simulink model "PoLiFirstPrototipe"  (Simulink 7.9)
settings: Solver=ode45  StartTime=0.0  StopTime=10.0  RelTol=1e-3
undefined symbols (not defined in the file or in its folder): sigbuilder_block
settings Model: Creator=lanalfa  LastModifiedBy=lanalfa

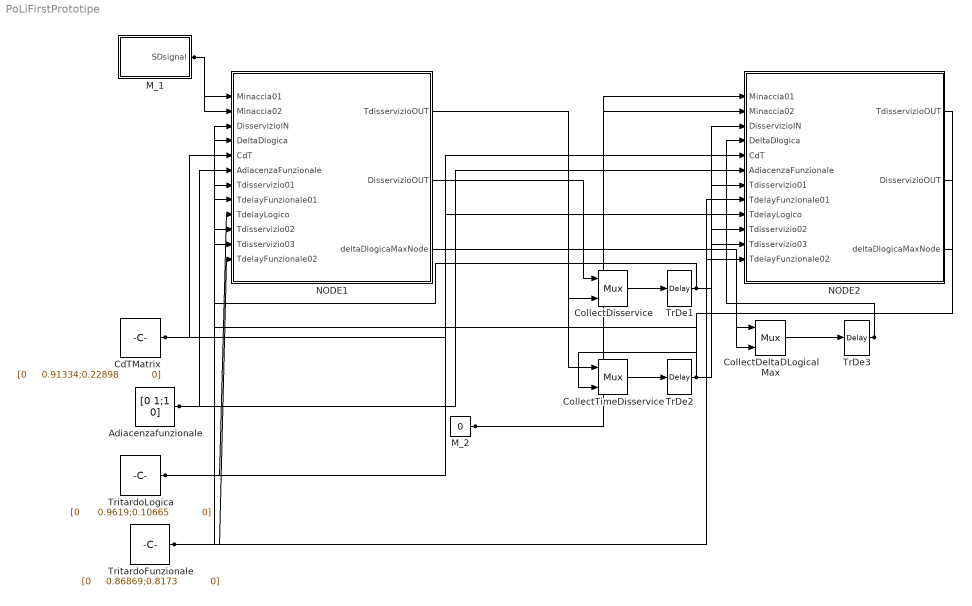
== system PoLiFirstPrototipe ==
  Adiacenzafunzionale : Constant  Value="[0  1;1  0]"
  CdTMatrix : Constant  Value="[0     0.91334;0.22898           0]"
  CollectDeltaDLogicalMax : Mux  Inputs=[-1 -1]
  CollectDisservice : Mux  Inputs=[-1 -1]
  CollectTimeDisservice : Mux  Inputs=[-1 -1]
  M_1 : Subsystem  Tag=STV Subsys  LoadFcn=sigbuilder_block('load');  StartFcn=sigbuilder_block('start');  StopFcn=sigbuilder_block('stop');  ClipboardFcn=sigbuilder_block('clipboard');  mask(Sigbuilder block){}
      mask init:
      | if ~strcmp(get_param(bdroot(gcb),'SimulationStatus'),'stopped'),tuvar = sigbuilder_block('maskInit'); end
      settings: CopyFcn=sigbuilder_block('copy');  DeleteFcn=sigbuilder_block('delete');  ModelCloseFcn=sigbuilder_block('modelClose');  PreSaveFcn=sigbuilder_block('preSave');  NameChangeFcn=sigbuilder_block('namechange');  OpenFcn=sigbuilder_block('open',[50.25 50.25 519.75 399.75 ]);  CloseFcn=sigbuilder_block('close');
      mask Display: plot(0, 0, 100, 100,[2, 2, 32, 32, 2], [68, 8, 8, 68, 68],[32, 2], [38, 38], [32, 19, 2],[53, 60, 44], [32, 17, 17, 2],[16, 16, 31, 31]);txt = getActiveGroup(gcbh);text(2, 100, txt,'verticalAlignment', 'top');
  M_2 : Constant  Value=0
  NODE1 : Subsystem
  NODE2 : Subsystem
  TrDe1 : TransportDelay  DelayTime=0.081472
  TrDe2 : TransportDelay  DelayTime=0.081472
  TrDe3 : TransportDelay  DelayTime=0.081472
  TritardoFunzionale : Constant  Value="[0     0.86869;0.8173           0]"
  TritardoLogica : Constant  Value="[0      0.9619;0.10665           0]"
  wires:
  M_1/1(SDsignal) -> NODE1/1(Minaccia01), NODE1/2(Minaccia02)
  M_2/1 -> NODE2/1(Minaccia01), NODE2/2(Minaccia02)
  CollectDisservice/1 -> TrDe1/1
  CollectTimeDisservice/1 -> TrDe2/1
  CollectDeltaDLogicalMax/1 -> TrDe3/1
  CdTMatrix/1 -> NODE1/5(CdT), NODE2/5(CdT)
  Adiacenzafunzionale/1 -> NODE1/6(AdiacenzaFunzionale), NODE2/6(AdiacenzaFunzionale)
  TritardoLogica/1 -> NODE1/9(TdelayLogico), NODE2/9(TdelayLogico)
  TritardoFunzionale/1 -> NODE1/8(TdelayFunzionale01), NODE1/12(TdelayFunzionale02), NODE2/8(TdelayFunzionale01), NODE2/12(TdelayFunzionale02)
  TrDe1/1 -> NODE1/3(DisservizioIN), NODE2/3(DisservizioIN)
  TrDe2/1 -> NODE1/7(Tdisservizio01), NODE1/10(Tdisservizio02), NODE1/11(Tdisservizio03), NODE2/7(Tdisservizio01), NODE2/10(Tdisservizio02), NODE2/11(Tdisservizio03)
  TrDe3/1 -> NODE1/4(DeltaDlogica), NODE2/4(DeltaDlogica)
  NODE1/1(TdisservizioOUT) -> CollectTimeDisservice/1
  NODE1/2(DisservizioOUT) -> CollectDisservice/1
  NODE1/3(deltaDlogicaMaxNode) -> CollectDeltaDLogicalMax/1
  NODE2/1(TdisservizioOUT) -> CollectTimeDisservice/2
  NODE2/2(DisservizioOUT) -> CollectDisservice/2
  NODE2/3(deltaDlogicaMaxNode) -> CollectDeltaDLogicalMax/2

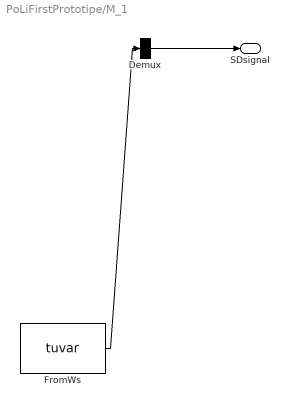
== system PoLiFirstPrototipe/M_1 ==
  Demux : Demux  Tag=STV Demux  Outputs=1
  FromWs : FromWorkspace  Tag=STV FromWs  VariableName=tuvar  SampleTime=0  SigBuilderData=DataTag0  VnvData=DataTag1
      SigBuilderData=|
      | dataSet.timeRange = [0 24]
      | dataSet.name = 'Group 1'
      | sbobj.Name = 'Signal Builder'
      | sbobj.Groups.Name = 'Group 1'
      | sbobj.Groups.Signals.Name = 'SDsignal'
      | sbobj.Groups.Signals.XData = [0 1 1 4 4 8 8 10 10 24]
      | sbobj.Groups.Signals.YData = [0 0 1 1 0 0 0.5 0.5 0 0]
      | sbobj.Groups.TimeRange = [0 24]
  SDsignal : Outport  Tag=STV Outport
  wires:
  FromWs/1 -> Demux/1
  Demux/1 -> SDsignal/1

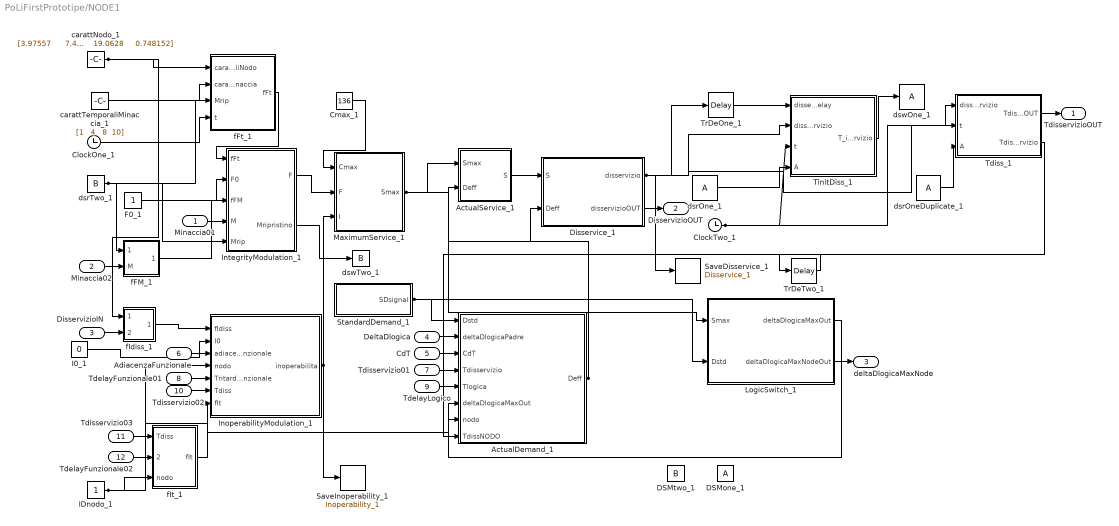
== system PoLiFirstPrototipe/NODE1 ==
  Minaccia01 : Inport
  Minaccia02 : Inport  Port=2
  DisservizioIN : Inport  Port=3
  DeltaDlogica : Inport  Port=4
  CdT : Inport  Port=5
  AdiacenzaFunzionale : Inport  Port=6
  Tdisservizio01 : Inport  Port=7
  TdelayFunzionale01 : Inport  Port=8
  TdelayLogico : Inport  Port=9
  Tdisservizio02 : Inport  Port=10
  Tdisservizio03 : Inport  Port=11
  TdelayFunzionale02 : Inport  Port=12
  ActualDemand_1 : MATLAB Function  TreatAsAtomicUnit=on
  ActualService_1 : MATLAB Function  TreatAsAtomicUnit=on
  ClockOne_1 : Clock
  ClockTwo_1 : Clock
  Cmax_1 : Constant  Value=136
  DSMone_1 : DataStoreMemory
  DSMtwo_1 : DataStoreMemory  DataStoreName=B
  Disservice_1 : MATLAB Function  TreatAsAtomicUnit=on
  F0_1 : Constant
  I0_1 : Constant  Value=0
  IDnodo_1 : Constant
  InoperabilityModulation_1 : MATLAB Function  TreatAsAtomicUnit=on
  IntegrityModulation_1 : MATLAB Function  TreatAsAtomicUnit=on
  LogicSwitch_1 : MATLAB Function  TreatAsAtomicUnit=on
  MaximumService_1 : MATLAB Function  TreatAsAtomicUnit=on
  SaveDisservice_1 : ToWorkspace  VariableName=Disservice_1  SampleTime=-1
  SaveInoperability_1 : ToWorkspace  VariableName=Inoperability_1  SampleTime=-1
  StandardDemand_1 : Subsystem  Tag=STV Subsys  LoadFcn=sigbuilder_block('load');  StartFcn=sigbuilder_block('start');  StopFcn=sigbuilder_block('stop');  ClipboardFcn=sigbuilder_block('clipboard');  mask(Sigbuilder block){}
      mask init:
      | if ~strcmp(get_param(bdroot(gcb),'SimulationStatus'),'stopped'),tuvar = sigbuilder_block('maskInit'); end
      settings: CopyFcn=sigbuilder_block('copy');  DeleteFcn=sigbuilder_block('delete');  ModelCloseFcn=sigbuilder_block('modelClose');  PreSaveFcn=sigbuilder_block('preSave');  NameChangeFcn=sigbuilder_block('namechange');  OpenFcn=sigbuilder_block('open',[50.25 50.25 519.75 399.75 ]);  CloseFcn=sigbuilder_block('close');
      mask Display: plot(0, 0, 100, 100,[2, 2, 32, 32, 2], [68, 8, 8, 68, 68],[32, 2], [38, 38], [32, 19, 2],[53, 60, 44], [32, 17, 17, 2],[16, 16, 31, 31]);txt = getActiveGroup(gcbh);text(2, 100, txt,'verticalAlignment', 'top');
  Tdiss_1 : MATLAB Function  TreatAsAtomicUnit=on
  TinitDiss_1 : MATLAB Function  TreatAsAtomicUnit=on
  TrDeOne_1 : TransportDelay  DelayTime=0.081472
  TrDeTwo_1 : TransportDelay  DelayTime=0.081472
  carattNodo_1 : Constant  Value="[3.97557      7.46916      12.6848      19.0628     0.748152]"
  carattTemporaliMinaccia_1 : Constant  Value="[1   4   8  10]"
  dsrOneDuplicate_1 : DataStoreRead
  dsrOne_1 : DataStoreRead
  dsrTwo_1 : DataStoreRead  DataStoreName=B
  dswOne_1 : DataStoreWrite
  dswTwo_1 : DataStoreWrite  DataStoreName=B
  fFM_1 : MATLAB Function  TreatAsAtomicUnit=on
  fFt_1 : MATLAB Function  TreatAsAtomicUnit=on
  fIdiss_1 : MATLAB Function  TreatAsAtomicUnit=on
  fIt_1 : MATLAB Function  TreatAsAtomicUnit=on
  TdisservizioOUT : Outport
  DisservizioOUT : Outport  Port=2
  deltaDlogicaMaxNode : Outport  Port=3
  wires:
  carattNodo_1/1 -> fFt_1/1(carattTemporaliNodo), fIdiss_1/1(parameters)
  carattTemporaliMinaccia_1/1 -> fFt_1/2(carattTemporaliMinaccia)
  ClockOne_1/1 -> fFt_1/4(t)
  fFt_1/1(fFt) -> IntegrityModulation_1/1(fFt)
  dsrTwo_1/1 -> fFt_1/3(Mrip), IntegrityModulation_1/5(Mrip), fFM_1/1(Mrip)
  F0_1/1 -> IntegrityModulation_1/2(F0)
  fFM_1/1(fFM) -> IntegrityModulation_1/3(fFM)
  IntegrityModulation_1/1(F) -> MaximumService_1/2(F)
  IntegrityModulation_1/2(Mripristino) -> dswTwo_1/1
  MaximumService_1/1(Smax) -> ActualService_1/1(Smax), LogicSwitch_1/1(Smax)
  Cmax_1/1 -> MaximumService_1/1(Cmax)
  ActualService_1/1(S) -> Disservice_1/1(S)
  Disservice_1/1(disservizio) -> TinitDiss_1/2(disservizio), Tdiss_1/1(disservizio), TrDeOne_1/1, SaveDisservice_1/1
  TinitDiss_1/1(T_inizio_disservizio) -> dswOne_1/1
  Tdiss_1/2(Tdisservizio) -> TrDeTwo_1/1
  TrDeOne_1/1 -> TinitDiss_1/1(disservizioDelay)
  ClockTwo_1/1 -> TinitDiss_1/3(t), Tdiss_1/2(t)
  dsrOne_1/1 -> TinitDiss_1/4(A)
  dsrOneDuplicate_1/1 -> Tdiss_1/3(A)
  InoperabilityModulation_1/1(inoperabilita) -> MaximumService_1/3(I), SaveInoperability_1/1
  ActualDemand_1/1(Deff) -> ActualService_1/2(Deff), Disservice_1/2(Deff)
  LogicSwitch_1/1(deltaDlogicaMaxOut) -> ActualDemand_1/6(deltaDlogicaMaxOut)
  fIdiss_1/1(fIdiss) -> InoperabilityModulation_1/1(fIdiss)
  I0_1/1 -> InoperabilityModulation_1/2(I0)
  fIt_1/1(fIt) -> InoperabilityModulation_1/7(fIt)
  IDnodo_1/1 -> InoperabilityModulation_1/4(nodo), ActualDemand_1/7(nodo), fIt_1/3(nodo)
  StandardDemand_1/1(SDsignal) -> ActualDemand_1/1(Dstd), LogicSwitch_1/2(Dstd)
  TrDeTwo_1/1 -> ActualDemand_1/8(TdissNODO)
  Tdiss_1/1(TdisservizioOUT) -> TdisservizioOUT/1
  Disservice_1/2(disservizioOUT) -> DisservizioOUT/1
  Minaccia01/1 -> IntegrityModulation_1/4(M)
  Minaccia02/1 -> fFM_1/2(M)
  DisservizioIN/1 -> fIdiss_1/2(DisservizioIN)
  DeltaDlogica/1 -> ActualDemand_1/2(deltaDlogicaPadre)
  CdT/1 -> ActualDemand_1/3(CdT)
  AdiacenzaFunzionale/1 -> InoperabilityModulation_1/3(adiacenzaFunzionale)
  LogicSwitch_1/2(deltaDlogicaMaxNodeOut) -> deltaDlogicaMaxNode/1
  Tdisservizio01/1 -> ActualDemand_1/4(Tdisservizio)
  TdelayFunzionale01/1 -> InoperabilityModulation_1/5(TritardoFunzionale)
  TdelayLogico/1 -> ActualDemand_1/5(Tlogica)
  Tdisservizio02/1 -> InoperabilityModulation_1/6(Tdiss)
  Tdisservizio03/1 -> fIt_1/1(Tdiss)
  TdelayFunzionale02/1 -> fIt_1/2(TritardoFunzionale)

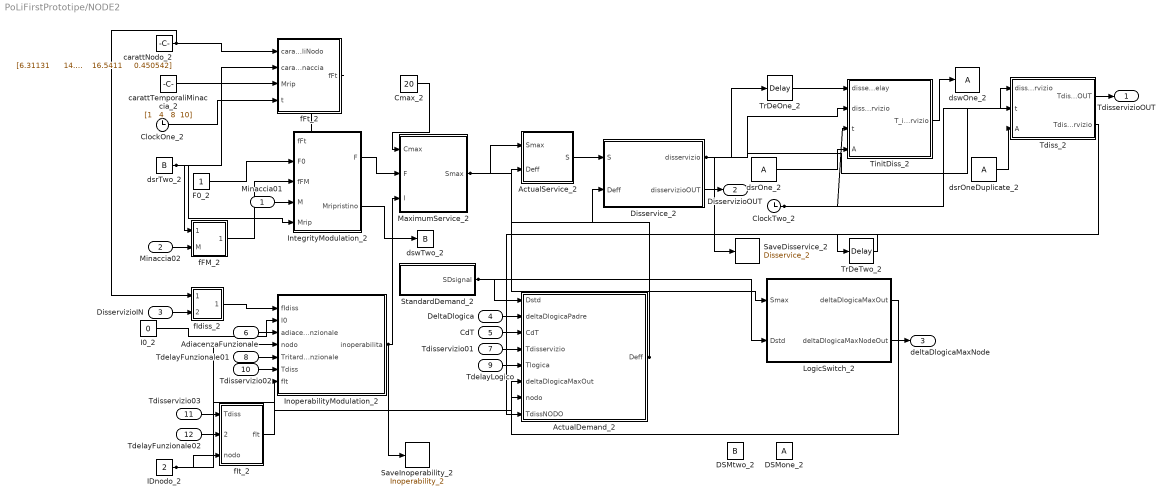
== system PoLiFirstPrototipe/NODE2 ==
  Minaccia01 : Inport
  Minaccia02 : Inport  Port=2
  DisservizioIN : Inport  Port=3
  DeltaDlogica : Inport  Port=4
  CdT : Inport  Port=5
  AdiacenzaFunzionale : Inport  Port=6
  Tdisservizio01 : Inport  Port=7
  TdelayFunzionale01 : Inport  Port=8
  TdelayLogico : Inport  Port=9
  Tdisservizio02 : Inport  Port=10
  Tdisservizio03 : Inport  Port=11
  TdelayFunzionale02 : Inport  Port=12
  ActualDemand_2 : MATLAB Function  TreatAsAtomicUnit=on
  ActualService_2 : MATLAB Function  TreatAsAtomicUnit=on
  ClockOne_2 : Clock
  ClockTwo_2 : Clock
  Cmax_2 : Constant  Value=20
  DSMone_2 : DataStoreMemory
  DSMtwo_2 : DataStoreMemory  DataStoreName=B
  Disservice_2 : MATLAB Function  TreatAsAtomicUnit=on
  F0_2 : Constant
  I0_2 : Constant  Value=0
  IDnodo_2 : Constant  Value=2
  InoperabilityModulation_2 : MATLAB Function  TreatAsAtomicUnit=on
  IntegrityModulation_2 : MATLAB Function  TreatAsAtomicUnit=on
  LogicSwitch_2 : MATLAB Function  TreatAsAtomicUnit=on
  MaximumService_2 : MATLAB Function  TreatAsAtomicUnit=on
  SaveDisservice_2 : ToWorkspace  VariableName=Disservice_2  SampleTime=-1
  SaveInoperability_2 : ToWorkspace  VariableName=Inoperability_2  SampleTime=-1
  StandardDemand_2 : Subsystem  Tag=STV Subsys  LoadFcn=sigbuilder_block('load');  StartFcn=sigbuilder_block('start');  StopFcn=sigbuilder_block('stop');  ClipboardFcn=sigbuilder_block('clipboard');  mask(Sigbuilder block){}
      mask init:
      | if ~strcmp(get_param(bdroot(gcb),'SimulationStatus'),'stopped'),tuvar = sigbuilder_block('maskInit'); end
      settings: CopyFcn=sigbuilder_block('copy');  DeleteFcn=sigbuilder_block('delete');  ModelCloseFcn=sigbuilder_block('modelClose');  PreSaveFcn=sigbuilder_block('preSave');  NameChangeFcn=sigbuilder_block('namechange');  OpenFcn=sigbuilder_block('open',[50.25 50.25 519.75 399.75 ]);  CloseFcn=sigbuilder_block('close');
      mask Display: plot(0, 0, 100, 100,[2, 2, 32, 32, 2], [68, 8, 8, 68, 68],[32, 2], [38, 38], [32, 19, 2],[53, 60, 44], [32, 17, 17, 2],[16, 16, 31, 31]);txt = getActiveGroup(gcbh);text(2, 100, txt,'verticalAlignment', 'top');
  Tdiss_2 : MATLAB Function  TreatAsAtomicUnit=on
  TinitDiss_2 : MATLAB Function  TreatAsAtomicUnit=on
  TrDeOne_2 : TransportDelay  DelayTime=0.081472
  TrDeTwo_2 : TransportDelay  DelayTime=0.081472
  carattNodo_2 : Constant  Value="[6.31131      14.4476      15.6979      16.5411     0.450542]"
  carattTemporaliMinaccia_2 : Constant  Value="[1   4   8  10]"
  dsrOneDuplicate_2 : DataStoreRead
  dsrOne_2 : DataStoreRead
  dsrTwo_2 : DataStoreRead  DataStoreName=B
  dswOne_2 : DataStoreWrite
  dswTwo_2 : DataStoreWrite  DataStoreName=B
  fFM_2 : MATLAB Function  TreatAsAtomicUnit=on
  fFt_2 : MATLAB Function  TreatAsAtomicUnit=on
  fIdiss_2 : MATLAB Function  TreatAsAtomicUnit=on
  fIt_2 : MATLAB Function  TreatAsAtomicUnit=on
  TdisservizioOUT : Outport
  DisservizioOUT : Outport  Port=2
  deltaDlogicaMaxNode : Outport  Port=3
  wires:
  carattNodo_2/1 -> fFt_2/1(carattTemporaliNodo), fIdiss_2/1(parameters)
  carattTemporaliMinaccia_2/1 -> fFt_2/2(carattTemporaliMinaccia)
  ClockOne_2/1 -> fFt_2/4(t)
  fFt_2/1(fFt) -> IntegrityModulation_2/1(fFt)
  dsrTwo_2/1 -> fFt_2/3(Mrip), IntegrityModulation_2/5(Mrip), fFM_2/1(Mrip)
  F0_2/1 -> IntegrityModulation_2/2(F0)
  fFM_2/1(fFM) -> IntegrityModulation_2/3(fFM)
  IntegrityModulation_2/1(F) -> MaximumService_2/2(F)
  IntegrityModulation_2/2(Mripristino) -> dswTwo_2/1
  MaximumService_2/1(Smax) -> ActualService_2/1(Smax), LogicSwitch_2/1(Smax)
  Cmax_2/1 -> MaximumService_2/1(Cmax)
  ActualService_2/1(S) -> Disservice_2/1(S)
  Disservice_2/1(disservizio) -> TinitDiss_2/2(disservizio), Tdiss_2/1(disservizio), TrDeOne_2/1, SaveDisservice_2/1
  TinitDiss_2/1(T_inizio_disservizio) -> dswOne_2/1
  Tdiss_2/2(Tdisservizio) -> TrDeTwo_2/1
  TrDeOne_2/1 -> TinitDiss_2/1(disservizioDelay)
  ClockTwo_2/1 -> TinitDiss_2/3(t), Tdiss_2/2(t)
  dsrOne_2/1 -> TinitDiss_2/4(A)
  dsrOneDuplicate_2/1 -> Tdiss_2/3(A)
  InoperabilityModulation_2/1(inoperabilita) -> MaximumService_2/3(I), SaveInoperability_2/1
  ActualDemand_2/1(Deff) -> ActualService_2/2(Deff), Disservice_2/2(Deff)
  LogicSwitch_2/1(deltaDlogicaMaxOut) -> ActualDemand_2/6(deltaDlogicaMaxOut)
  fIdiss_2/1(fIdiss) -> InoperabilityModulation_2/1(fIdiss)
  I0_2/1 -> InoperabilityModulation_2/2(I0)
  fIt_2/1(fIt) -> InoperabilityModulation_2/7(fIt)
  IDnodo_2/1 -> InoperabilityModulation_2/4(nodo), ActualDemand_2/7(nodo), fIt_2/3(nodo)
  StandardDemand_2/1(SDsignal) -> ActualDemand_2/1(Dstd), LogicSwitch_2/2(Dstd)
  TrDeTwo_2/1 -> ActualDemand_2/8(TdissNODO)
  Tdiss_2/1(TdisservizioOUT) -> TdisservizioOUT/1
  Disservice_2/2(disservizioOUT) -> DisservizioOUT/1
  Minaccia01/1 -> IntegrityModulation_2/4(M)
  Minaccia02/1 -> fFM_2/2(M)
  DisservizioIN/1 -> fIdiss_2/2(DisservizioIN)
  DeltaDlogica/1 -> ActualDemand_2/2(deltaDlogicaPadre)
  CdT/1 -> ActualDemand_2/3(CdT)
  AdiacenzaFunzionale/1 -> InoperabilityModulation_2/3(adiacenzaFunzionale)
  LogicSwitch_2/2(deltaDlogicaMaxNodeOut) -> deltaDlogicaMaxNode/1
  Tdisservizio01/1 -> ActualDemand_2/4(Tdisservizio)
  TdelayFunzionale01/1 -> InoperabilityModulation_2/5(TritardoFunzionale)
  TdelayLogico/1 -> ActualDemand_2/5(Tlogica)
  Tdisservizio02/1 -> InoperabilityModulation_2/6(Tdiss)
  Tdisservizio03/1 -> fIt_2/1(Tdiss)
  TdelayFunzionale02/1 -> fIt_2/2(TritardoFunzionale)

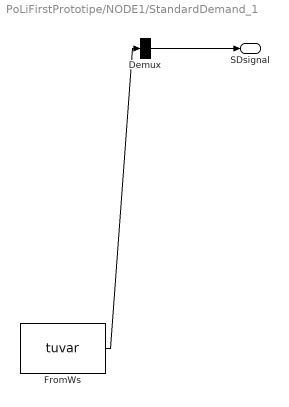
== system PoLiFirstPrototipe/NODE1/StandardDemand_1 ==
  Demux : Demux  Tag=STV Demux  Outputs=1
  FromWs : FromWorkspace  Tag=STV FromWs  VariableName=tuvar  SampleTime=0  SigBuilderData=DataTag2  VnvData=DataTag3
      SigBuilderData=|
      | dataSet.timeRange = [0 24]
      | dataSet.name = 'Group 1'
      | sbobj.Name = 'Signal Builder'
      | sbobj.Groups.Name = 'Group 1'
      | sbobj.Groups.Signals.Name = 'SDsignal'
      | sbobj.Groups.Signals.XData = [0 0.5 1 1.5 2 2.5 3 3.5 4 4.5 5 5.5 6 6.5 7 7.5 8 8.5 9 9.5 10 10.5 11 11.5 12 12.5 13 13.5 14 14.5 15 15.5 16 16.5 17 17.5 18 18.5 19 19.5 20 20.5 21 21.5 22 22.5 23 23.5 24]
      | sbobj.Groups.Signals.YData = [11.7808835651 122.73450492 61.6241133881 4.7751592129 3.99938168056 69.9889117737 116.703457947 11.4599685743 5.50903001057 131.143211714 8.97691830497 32.9473422413 82.6571253434 112.718610458 131.670732893 129.720690874 24.0097353475 92.8744707117 131.315333052 84.1080498354 27.8528134454 69.3920421728 48.1014306249 33.3626112504 43.5604359479 113.884804014 68.2224889304 89.7075411734 105.561576229 101.307064298 40.9255657187 5.53636617206 117.147075775 100.978877439 101.41762366 102.880604253 88.4022078261 101.852595315 71.6327165492 23.0073066061 61.2375892724 97.1258934404 33.4928431781 58.7762568614 128.662783861 30.0332567061 118.332755648 72.1628728161 90.1513203618]
      | sbobj.Groups.TimeRange = [0 24]
  SDsignal : Outport  Tag=STV Outport
  wires:
  FromWs/1 -> Demux/1
  Demux/1 -> SDsignal/1

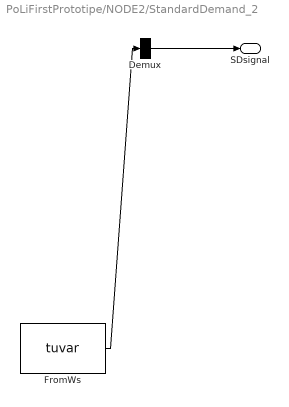
== system PoLiFirstPrototipe/NODE2/StandardDemand_2 ==
  Demux : Demux  Tag=STV Demux  Outputs=1
  FromWs : FromWorkspace  Tag=STV FromWs  VariableName=tuvar  SampleTime=0  SigBuilderData=DataTag4  VnvData=DataTag5
      SigBuilderData=|
      | dataSet.timeRange = [0 24]
      | dataSet.name = 'Group 1'
      | sbobj.Name = 'Signal Builder'
      | sbobj.Groups.Name = 'Group 1'
      | sbobj.Groups.Signals.Name = 'SDsignal'
      | sbobj.Groups.Signals.XData = [0 0.5 1 1.5 2 2.5 3 3.5 4 4.5 5 5.5 6 6.5 7 7.5 8 8.5 9 9.5 10 10.5 11 11.5 12 12.5 13 13.5 14 14.5 15 15.5 16 16.5 17 17.5 18 18.5 19 19.5 20 20.5 21 21.5 22 22.5 23 23.5 24]
      | sbobj.Groups.Signals.YData = [7.35281507549 14.4300356227 0.849863291314 16.8477383664 0.856661035141 3.99439062222 11.5647743475 4.15585340881 6.88518601687 3.01741388262 6.42529690284 5.1373506375 6.89044219645 5.87907823961 14.4615403008 18.0573643753 6.10342754048 0.995559023233 11.2251128069 4.68966423702 16.2625479089 11.0882759858 5.81270338284 14.47949846 6.89803992052 17.6200463688 0.805120829678 8.2946449804 4.97465881389 9.8808589667 2.18193494928 9.05568940072 17.0141198888 3.18565488033 3.71430347862 1.41472753626 16.0680949914 7.67910647707 12.9668098587 8.29471817695 1.6561267234 4.85599541779 12.3910830605 18.4829142087 9.38404893982 1.31978631542 8.62352678256 19.76195861 16.7563538361]
      | sbobj.Groups.TimeRange = [0 24]
  SDsignal : Outport  Tag=STV Outport
  wires:
  FromWs/1 -> Demux/1
  Demux/1 -> SDsignal/1

== matlab function NODE1/fFM_1 ==
  data: Mrip input double; fFM output double; M input double
function fFM = f(Mrip,M)

% Function description:

% This function ....

% INPUT
% ...

% OUTPUT
% ...



%Funzione di modulazione dell'integrità funzionale in intensità retta con coefficiente=1
fFM=[0,0];
fFM(1)=M*1; %modulazione in intensità, %modulazione in intesità della minaccia FM=[0 a 1]
fFM(2)=Mrip*1; %modulazione in intensità, da usare solo per il recupero di integrità,cioè quando M=0;

== matlab function NODE1/fFt_1 ==
  data: carattTemporaliNodo input double; fFt output double; carattTemporaliMinaccia input double; Mrip input double; t input double
function fFt = f(carattTemporaliNodo,carattTemporaliMinaccia,Mrip,t)

% Function description:

% This function ....

% INPUT
% ...

% OUTPUT
% ...

%Funzione di modulazione dell'integrità funzionale nel tempo, nel caso di
%due minaccie differenti per inizio attacco nel tempo.

Tbuffer=carattTemporaliNodo(1);
Tpropagazione=carattTemporaliNodo(2);
TorganizzazioneMax=carattTemporaliNodo(3);
TripristinoMax=carattTemporaliNodo(4);
TinizioM1=carattTemporaliMinaccia(1);  %da impostare manualmente nelle descrizione minaccia
TfineM1=carattTemporaliMinaccia(2); %da impostare manualmente nelle descrizione minaccia
TinizioM2=carattTemporaliMinaccia(3); %da impostare manualmente nelle descrizione minaccia
TfineM2=carattTemporaliMinaccia(4); %da impostare manualmente nelle descrizione minaccia
Torganizzazione=Mrip*TorganizzazioneMax;
Tripristino=TripristinoMax*Mrip; %in realtà sarebbe Tripristino=TripristinoMax*M; ma così M mi annulla il ripristino a fine minaccia, uso minaccia salvata  
tauRipristino=Tripristino/5; %controllare se vale anche per nodo non trasporto
tauPropagazione=Tpropagazione/5; %controllare se vale anche per nodo non trasporto
t0=TinizioM1+Tbuffer;
t1=t0+Tpropagazione;
t2o=t1+Torganizzazione;
t2m=TfineM1;
if t2m>=t2o %chiarire cosa succede se M=0 ma non ancora organizzato (t2o>t2m) e quindi cosa fa integrità funzionale
    t2=t2m;
else t2=t2o;
end
t3=t2+Tripristino;
t4=TinizioM2+Tbuffer;
t5=t4+Tpropagazione;
t6m=TfineM2;
t6o=t5+Torganizzazione; 
if t6m>=t6o
    t6=t6m;
else t6=t6o;
end
t7=t6+Tripristino;

if t<t0
    fFt=0;
elseif t>=t0 && t<t1 
        fFt=1-exp(-(t-t0)/tauPropagazione);
elseif t>=t1 && t<t2
        fFt=1;
elseif t>=t2 && t<t3 
        fFt=exp(-(t-t2)/tauRipristino);  
elseif t>=t4 && t<t5
        fFt=1-exp(-(t-t4)/tauPropagazione);
elseif t>=t5 && t<t6
        fFt=1;
elseif t>=t6 && t<t7
        fFt=exp(-(t-t6)/tauRipristino);  
else fFt=0;
end

== matlab function NODE1/IntegrityModulation_1 ==
  data: fFt input double; F output double; F0 input double; fFM input double; M input double; Mrip input double; Mripristino output double
function [F,Mripristino] = f(fFt,F0,fFM,M,Mrip)

% Function description:

% This function ....

% INPUT
% ...

% OUTPUT
% ...


% Codice con valutazione solo in intesità, non nel tempo.
% fFM=M*FM; %modulazione in intensità
% fFt=1;
% i=F0-fFM*fFt;
%
% if i<0
%     F=0;
% else
%     F=i;
% end

% Codice con valutazione in intensità e tempo con doppia attacco da parte della minaccia

% Modifica per avere ripristino a fine minaccia, in realtà sarebbe sempre i=F0-fFM*fFt

if M>0
    i=F0-fFM(1)*fFt;
    Mripristino=M;
else i=F0-fFM(2)*fFt; %fFM(2) è quella usata solo per il ripristino di integrità perchè M=0;
    Mripristino=Mrip;
end

if i<0
    F=0;
else
    F=i;
end

== matlab function NODE1/MaximumService_1 ==
  data: Cmax input double; Smax output double; F input double; I input double
function Smax = f(Cmax,F,I)

% Function description:

% This function ....

% INPUT
% ...

% OUTPUT
% ...


Smax=F*(1-I)*Cmax;

end

== matlab function NODE1/ActualService_1 ==
  data: Smax input double; S output double; Deff input double
function S = f(Smax,Deff)

% Function description:

% This function ....

% INPUT
% ...

% OUTPUT
% ...

if Deff>Smax
    S=Smax;
else
    S=Deff;
end

== matlab function NODE1/Disservice_1 ==
  data: S input double; disservizio output double; Deff input double; disservizioOUT output double
function [disservizio,disservizioOUT ] = f(S,Deff)

% Function description:

% This function ....

% INPUT
% ...

% OUTPUT
% ...

if Deff==0
    disservizio=0;
else
disservizio=(Deff-S)/Deff;

end

disservizioOUT=disservizio;

== matlab function NODE1/TinitDiss_1 ==
  data: disservizioDelay input double; T_inizio_disservizio output double; disservizio input double; t input double; A input double
function T_inizio_disservizio  = f(disservizioDelay,disservizio,t,A)

% Function description:

% This function ....

% INPUT
% ...

% OUTPUT
% ...

if disservizioDelay==0 && disservizio>0
    T_inizio_disservizio=t;
else T_inizio_disservizio=A;

end

% if disservizioDelay~=disservizio && disservizio>0
%     T_inizio_variazioneDiss=t;
% else T_inizio_variazioneDiss=B;
% end
%

== matlab function NODE1/Tdiss_1 ==
  data: disservizio input double; TdisservizioOUT output double; t input double; A input double; Tdisservizio output double
function [TdisservizioOUT,Tdisservizio]  = f(disservizio,t,A)

% Function description:

% This function ....

% INPUT
% ...

% OUTPUT
% ...


if disservizio==0
    Tdisservizio=0;
else
    Tdisservizio=t-A;
end
% if disservizio==0
%     TvariazioneDiss=0;
% else
%     TvariazioneDiss=t-B;
% end

TdisservizioOUT=Tdisservizio;

== matlab function NODE1/InoperabilityModulation_1 ==
  data: fIdiss input double; inoperabilita output double; I0 input double; adiacenzaFunzionale input double; nodo input double; TritardoFunzionale input double; Tdiss input double; fIt input double
function inoperabilita = f(fIdiss,I0,adiacenzaFunzionale,nodo,TritardoFunzionale,Tdiss,fIt)

% Function description:

% This function ....

% INPUT
% ...

% OUTPUT
% ...


j=1;
disservizioTot=zeros(length(adiacenzaFunzionale),1);
for j=1:length(adiacenzaFunzionale)
    if adiacenzaFunzionale(j,nodo)==1 && Tdiss(j)>=TritardoFunzionale(j,nodo)
        disservizioTot(j,1)=fIdiss(1,j)*fIt(1,j);
        %disservizioTot(j,1)=fIdiss; se non voglio avere
        %modulazione nel tempo del trasferimento di disservizio in
        %inoperabilità
    else disservizioTot(j,1)=0;
    end
end

disservizioTotIN=sum(disservizioTot); % ho fatto somma, altro approccio prendere il max
i=I0+disservizioTotIN;

if i>1
    inoperabilita=1;
elseif i<=0
    inoperabilita=0;
else inoperabilita=i;
end

== matlab function NODE1/ActualDemand_1 ==
  data: Dstd input double; Deff output double; deltaDlogicaPadre input double; CdT input double; Tdisservizio input double; Tlogica input double; deltaDlogicaMaxOut input double; nodo input double; TdissNODO input double
function Deff= f(Dstd,deltaDlogicaPadre,CdT,Tdisservizio,Tlogica,deltaDlogicaMaxOut,nodo,TdissNODO)
 
% Function description:
 
% This function ....
 
% INPUT
% ...
 
% OUTPUT
% ...
 
 
j=1;
deltaDlogicaOUT=zeros(length(CdT),1);
deltaDlogicaIN=zeros(length(CdT),1);
 
 
for j=1:(length(CdT))
    if Tdisservizio(j)>=Tlogica(j,nodo) && CdT(j,nodo)>0
        deltaDlogicaIN(j,1)=CdT(j,nodo)*deltaDlogicaPadre(j);
    else
        deltaDlogicaIN(j,1)=0;
    end
    if TdissNODO>=Tlogica(nodo,j) && CdT(nodo,j)>0
          deltaDlogicaOUT(j,1)=CdT(nodo,j)*deltaDlogicaMaxOut;
    else
        deltaDlogicaOUT(j,1)=0;
    end
end
deltaDlogicaTotIN=sum(deltaDlogicaIN);
deltaDlogicaTotOut=sum(deltaDlogicaOUT);
 
 
Deff=Dstd+deltaDlogicaTotIN-deltaDlogicaTotOut;

== matlab function NODE1/LogicSwitch_1 ==
  data: Smax input double; deltaDlogicaMaxOut output double; Dstd input double; deltaDlogicaMaxNodeOut output double
function [deltaDlogicaMaxOut,deltaDlogicaMaxNodeOut] = f(Smax,Dstd)

% Function description:

% This function ....

% INPUT
% ...

% OUTPUT
% ...

deltaDlogicaMaxOut=Dstd-Smax;
if deltaDlogicaMaxOut<0
    deltaDlogicaMaxOut=0;
end

deltaDlogicaMaxNodeOut=deltaDlogicaMaxOut;

== matlab function NODE1/fIdiss_1 ==
  data: parameters input double; fIdiss output double; DisservizioIN input double
function fIdiss = f(parameters,DisservizioIN)

% Function description:

% This function ....

% INPUT
% ...

% OUTPUT
% ...


%Funzione di modulazion lineare con coefficiente angolare variabile,
fIdiss=zeros(1,length(DisservizioIN));
j=1;
for j=1:length(DisservizioIN)
    fIdiss(1,j)=DisservizioIN(j)*parameters(5);% modulazione in intensità
end

== matlab function NODE1/fIt_1 ==
  data: Tdiss input double; fIt output double; TritardoFunzionale input double; nodo input double
function fIt = f(Tdiss,TritardoFunzionale,nodo)

% Function description:

% This function ....

% INPUT
% ...

% OUTPUT
% ...

%funzione di modulazione dell'inoperabilità nel tempo
fIt=zeros(1,length(Tdiss));
j=1;
for j=1:length(Tdiss)
    tau=TritardoFunzionale(j,nodo)/5; %vedere se anche per i nodi non di trasporto vale questa tau!!!
    fIt(1,j)=1-exp(-(Tdiss(j)-TritardoFunzionale(j,nodo))/tau);%modulazione nel tempo
end

== matlab function NODE2/fFt_2 ==
  data: carattTemporaliNodo input double; fFt output double; carattTemporaliMinaccia input double; Mrip input double; t input double
function fFt = f(carattTemporaliNodo,carattTemporaliMinaccia,Mrip,t)

% Function description:

% This function ....

% INPUT
% ...

% OUTPUT
% ...

%Funzione di modulazione dell'integrità funzionale nel tempo, nel caso di
%due minaccie differenti per inizio attacco nel tempo.

Tbuffer=carattTemporaliNodo(1);
Tpropagazione=carattTemporaliNodo(2);
TorganizzazioneMax=carattTemporaliNodo(3);
TripristinoMax=carattTemporaliNodo(4);
TinizioM1=carattTemporaliMinaccia(1);  %da impostare manualmente nelle descrizione minaccia
TfineM1=carattTemporaliMinaccia(2); %da impostare manualmente nelle descrizione minaccia
TinizioM2=carattTemporaliMinaccia(3); %da impostare manualmente nelle descrizione minaccia
TfineM2=carattTemporaliMinaccia(4); %da impostare manualmente nelle descrizione minaccia
Torganizzazione=Mrip*TorganizzazioneMax;
Tripristino=TripristinoMax*Mrip; %in realtà sarebbe Tripristino=TripristinoMax*M; ma così M mi annulla il ripristino a fine minaccia, uso minaccia salvata  
tauRipristino=Tripristino/5; %controllare se vale anche per nodo non trasporto
tauPropagazione=Tpropagazione/5; %controllare se vale anche per nodo non trasporto
t0=TinizioM1+Tbuffer;
t1=t0+Tpropagazione;
t2o=t1+Torganizzazione;
t2m=TfineM1;
if t2m>=t2o %chiarire cosa succede se M=0 ma non ancora organizzato (t2o>t2m) e quindi cosa fa integrità funzionale
    t2=t2m;
else t2=t2o;
end
t3=t2+Tripristino;
t4=TinizioM2+Tbuffer;
t5=t4+Tpropagazione;
t6m=TfineM2;
t6o=t5+Torganizzazione; 
if t6m>=t6o
    t6=t6m;
else t6=t6o;
end
t7=t6+Tripristino;

if t<t0
    fFt=0;
elseif t>=t0 && t<t1 
        fFt=1-exp(-(t-t0)/tauPropagazione);
elseif t>=t1 && t<t2
        fFt=1;
elseif t>=t2 && t<t3 
        fFt=exp(-(t-t2)/tauRipristino);  
elseif t>=t4 && t<t5
        fFt=1-exp(-(t-t4)/tauPropagazione);
elseif t>=t5 && t<t6
        fFt=1;
elseif t>=t6 && t<t7
        fFt=exp(-(t-t6)/tauRipristino);  
else fFt=0;
end

== matlab function NODE2/fFM_2 ==
  data: Mrip input double; fFM output double; M input double
function fFM = f(Mrip,M)

% Function description:

% This function ....

% INPUT
% ...

% OUTPUT
% ...



%Funzione di modulazione dell'integrità funzionale in intensità retta con coefficiente=1
fFM=[0,0];
fFM(1)=M*1; %modulazione in intensità, %modulazione in intesità della minaccia FM=[0 a 1]
fFM(2)=Mrip*1; %modulazione in intensità, da usare solo per il recupero di integrità,cioè quando M=0;

== matlab function NODE2/IntegrityModulation_2 ==
  data: fFt input double; F output double; F0 input double; fFM input double; M input double; Mrip input double; Mripristino output double
function [F,Mripristino] = f(fFt,F0,fFM,M,Mrip)

% Function description:

% This function ....

% INPUT
% ...

% OUTPUT
% ...


% Codice con valutazione solo in intesità, non nel tempo.
% fFM=M*FM; %modulazione in intensità
% fFt=1;
% i=F0-fFM*fFt;
%
% if i<0
%     F=0;
% else
%     F=i;
% end

% Codice con valutazione in intensità e tempo con doppia attacco da parte della minaccia

% Modifica per avere ripristino a fine minaccia, in realtà sarebbe sempre i=F0-fFM*fFt

if M>0
    i=F0-fFM(1)*fFt;
    Mripristino=M;
else i=F0-fFM(2)*fFt; %fFM(2) è quella usata solo per il ripristino di integrità perchè M=0;
    Mripristino=Mrip;
end

if i<0
    F=0;
else
    F=i;
end

== matlab function NODE2/MaximumService_2 ==
  data: Cmax input double; Smax output double; F input double; I input double
function Smax = f(Cmax,F,I)

% Function description:

% This function ....

% INPUT
% ...

% OUTPUT
% ...


Smax=F*(1-I)*Cmax;

end

== matlab function NODE2/ActualService_2 ==
  data: Smax input double; S output double; Deff input double
function S = f(Smax,Deff)

% Function description:

% This function ....

% INPUT
% ...

% OUTPUT
% ...

if Deff>Smax
    S=Smax;
else
    S=Deff;
end

== matlab function NODE2/Disservice_2 ==
  data: S input double; disservizio output double; Deff input double; disservizioOUT output double
function [disservizio,disservizioOUT ] = f(S,Deff)

% Function description:

% This function ....

% INPUT
% ...

% OUTPUT
% ...

if Deff==0
    disservizio=0;
else
disservizio=(Deff-S)/Deff;

end

disservizioOUT=disservizio;

== matlab function NODE2/TinitDiss_2 ==
  data: disservizioDelay input double; T_inizio_disservizio output double; disservizio input double; t input double; A input double
function T_inizio_disservizio  = f(disservizioDelay,disservizio,t,A)

% Function description:

% This function ....

% INPUT
% ...

% OUTPUT
% ...

if disservizioDelay==0 && disservizio>0
    T_inizio_disservizio=t;
else T_inizio_disservizio=A;

end

% if disservizioDelay~=disservizio && disservizio>0
%     T_inizio_variazioneDiss=t;
% else T_inizio_variazioneDiss=B;
% end
%

== matlab function NODE2/Tdiss_2 ==
  data: disservizio input double; TdisservizioOUT output double; t input double; A input double; Tdisservizio output double
function [TdisservizioOUT,Tdisservizio]  = f(disservizio,t,A)

% Function description:

% This function ....

% INPUT
% ...

% OUTPUT
% ...


if disservizio==0
    Tdisservizio=0;
else
    Tdisservizio=t-A;
end
% if disservizio==0
%     TvariazioneDiss=0;
% else
%     TvariazioneDiss=t-B;
% end

TdisservizioOUT=Tdisservizio;

== matlab function NODE2/InoperabilityModulation_2 ==
  data: fIdiss input double; inoperabilita output double; I0 input double; adiacenzaFunzionale input double; nodo input double; TritardoFunzionale input double; Tdiss input double; fIt input double
function inoperabilita = f(fIdiss,I0,adiacenzaFunzionale,nodo,TritardoFunzionale,Tdiss,fIt)

% Function description:

% This function ....

% INPUT
% ...

% OUTPUT
% ...


j=1;
disservizioTot=zeros(length(adiacenzaFunzionale),1);
for j=1:length(adiacenzaFunzionale)
    if adiacenzaFunzionale(j,nodo)==1 && Tdiss(j)>=TritardoFunzionale(j,nodo)
        disservizioTot(j,1)=fIdiss(1,j)*fIt(1,j);
        %disservizioTot(j,1)=fIdiss; se non voglio avere
        %modulazione nel tempo del trasferimento di disservizio in
        %inoperabilità
    else disservizioTot(j,1)=0;
    end
end

disservizioTotIN=sum(disservizioTot); % ho fatto somma, altro approccio prendere il max
i=I0+disservizioTotIN;

if i>1
    inoperabilita=1;
elseif i<=0
    inoperabilita=0;
else inoperabilita=i;
end

== matlab function NODE2/ActualDemand_2 ==
  data: Dstd input double; Deff output double; deltaDlogicaPadre input double; CdT input double; Tdisservizio input double; Tlogica input double; deltaDlogicaMaxOut input double; nodo input double; TdissNODO input double
function Deff= f(Dstd,deltaDlogicaPadre,CdT,Tdisservizio,Tlogica,deltaDlogicaMaxOut,nodo,TdissNODO)
 
% Function description:
 
% This function ....
 
% INPUT
% ...
 
% OUTPUT
% ...
 
 
j=1;
deltaDlogicaOUT=zeros(length(CdT),1);
deltaDlogicaIN=zeros(length(CdT),1);
 
 
for j=1:(length(CdT))
    if Tdisservizio(j)>=Tlogica(j,nodo) && CdT(j,nodo)>0
        deltaDlogicaIN(j,1)=CdT(j,nodo)*deltaDlogicaPadre(j);
    else
        deltaDlogicaIN(j,1)=0;
    end
    if TdissNODO>=Tlogica(nodo,j) && CdT(nodo,j)>0
          deltaDlogicaOUT(j,1)=CdT(nodo,j)*deltaDlogicaMaxOut;
    else
        deltaDlogicaOUT(j,1)=0;
    end
end
deltaDlogicaTotIN=sum(deltaDlogicaIN);
deltaDlogicaTotOut=sum(deltaDlogicaOUT);
 
 
Deff=Dstd+deltaDlogicaTotIN-deltaDlogicaTotOut;

== matlab function NODE2/LogicSwitch_2 ==
  data: Smax input double; deltaDlogicaMaxOut output double; Dstd input double; deltaDlogicaMaxNodeOut output double
function [deltaDlogicaMaxOut,deltaDlogicaMaxNodeOut] = f(Smax,Dstd)

% Function description:

% This function ....

% INPUT
% ...

% OUTPUT
% ...

deltaDlogicaMaxOut=Dstd-Smax;
if deltaDlogicaMaxOut<0
    deltaDlogicaMaxOut=0;
end

deltaDlogicaMaxNodeOut=deltaDlogicaMaxOut;

== matlab function NODE2/fIdiss_2 ==
  data: parameters input double; fIdiss output double; DisservizioIN input double
function fIdiss = f(parameters,DisservizioIN)

% Function description:

% This function ....

% INPUT
% ...

% OUTPUT
% ...


%Funzione di modulazion lineare con coefficiente angolare variabile,
fIdiss=zeros(1,length(DisservizioIN));
j=1;
for j=1:length(DisservizioIN)
    fIdiss(1,j)=DisservizioIN(j)*parameters(5);% modulazione in intensità
end

== matlab function NODE2/fIt_2 ==
  data: Tdiss input double; fIt output double; TritardoFunzionale input double; nodo input double
function fIt = f(Tdiss,TritardoFunzionale,nodo)

% Function description:

% This function ....

% INPUT
% ...

% OUTPUT
% ...

%funzione di modulazione dell'inoperabilità nel tempo
fIt=zeros(1,length(Tdiss));
j=1;
for j=1:length(Tdiss)
    tau=TritardoFunzionale(j,nodo)/5; %vedere se anche per i nodi non di trasporto vale questa tau!!!
    fIt(1,j)=1-exp(-(Tdiss(j)-TritardoFunzionale(j,nodo))/tau);%modulazione nel tempo
end
